simulink model "Model"  (R2019a)
settings: configuration reference "Configuration" (kept outside this file)
undefined symbols (not defined in the file): DiscIntNeverNeededParam
libraries: AP_Math x3, Quaternion x2
settings Model: Creator=zouji  LastModifiedBy=Bingo
settings ConfigSetRef: SourceName=Configuration  SourceLocation=Base Workspace

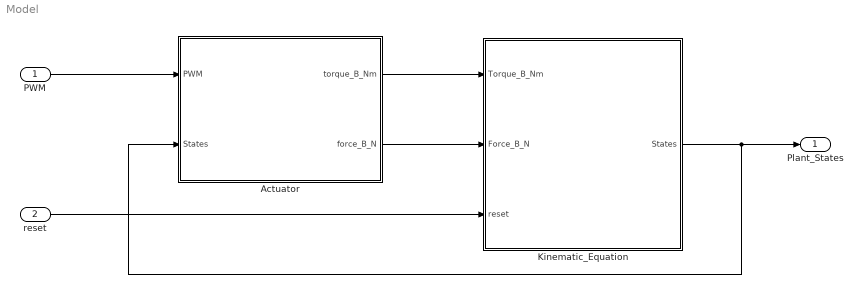
== system Model ==
  PWM : Inport
  reset : Inport  Port=2
  Actuator : Subsystem
  Kinematic_Equation : Subsystem
  Plant_States : Outport  OutDataTypeStr=Bus: Plant_States
  wires:
  Kinematic_Equation/1(States) -> Plant_States/1, Actuator/2(States)
  PWM/1 -> Actuator/1(PWM)
  Actuator/1(torque_B_Nm) -> Kinematic_Equation/1(Torque_B_Nm)
  Actuator/2(force_B_N) -> Kinematic_Equation/2(Force_B_N)
  reset/1 -> Kinematic_Equation/3(reset)

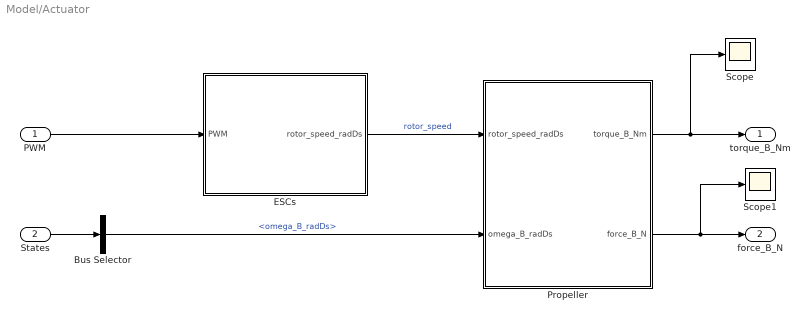
== system Model/Actuator ==
  PWM : Inport
  States : Inport  Port=2
  Bus Selector : BusSelector  OutputSignals=omega_B_radDs
  ESCs : Subsystem  mask{T=0.025, k=718.078, p=88.448}
  Propeller : Subsystem
  Scope : Scope
  Scope1 : Scope
  torque_B_Nm : Outport
  force_B_N : Outport  Port=2
  wires:
  PWM/1 -> ESCs/1(PWM)
  States/1 -> Bus Selector/1
  Bus Selector/1 -> Propeller/2(omega_B_radDs)  "<omega_B_radDs>"
  Propeller/1(torque_B_Nm) -> Scope/1, torque_B_Nm/1
  Propeller/2(force_B_N) -> Scope1/1, force_B_N/1
  ESCs/1(rotor_speed_radDs) -> Propeller/1(rotor_speed_radDs)  "rotor_speed"

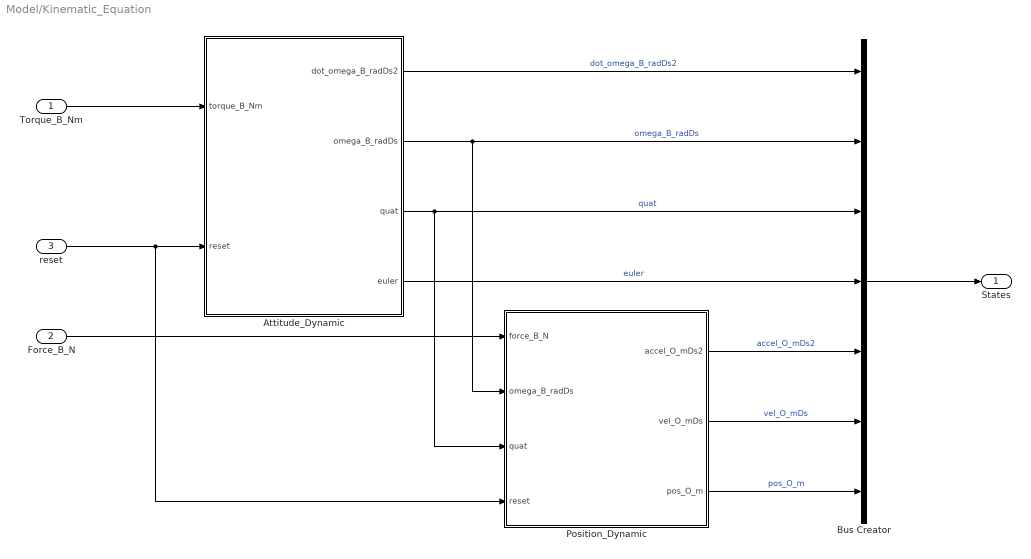
== system Model/Kinematic_Equation ==
  Torque_B_Nm : Inport
  Force_B_N : Inport  Port=2
  reset : Inport  Port=3
  Attitude_Dynamic : Subsystem  mask{Ixx=0.016, Iyy=0.016, Izz=0.0274}
  Bus Creator : BusCreator  Inputs=7
  Position_Dynamic : Subsystem  mask{mass=0.886}
  States : Outport
  wires:
  Torque_B_Nm/1 -> Attitude_Dynamic/1(torque_B_Nm)
  Force_B_N/1 -> Position_Dynamic/1(force_B_N)
  Attitude_Dynamic/2(omega_B_radDs) -> Bus Creator/2, Position_Dynamic/2(omega_B_radDs)  "omega_B_radDs"
  Attitude_Dynamic/3(quat) -> Bus Creator/3, Position_Dynamic/3(quat)  "quat"
  reset/1 -> Position_Dynamic/4(reset), Attitude_Dynamic/2(reset)
  Bus Creator/1 -> States/1
  Attitude_Dynamic/1(dot_omega_B_radDs2) -> Bus Creator/1  "dot_omega_B_radDs2"
  Attitude_Dynamic/4(euler) -> Bus Creator/4  "euler"
  Position_Dynamic/1(accel_O_mDs2) -> Bus Creator/5  "accel_O_mDs2"
  Position_Dynamic/2(vel_O_mDs) -> Bus Creator/6  "vel_O_mDs"
  Position_Dynamic/3(pos_O_m) -> Bus Creator/7  "pos_O_m"

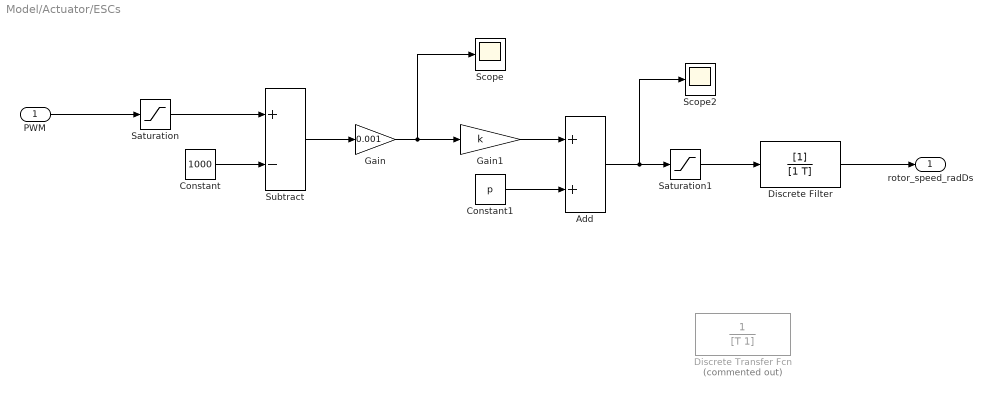
== system Model/Actuator/ESCs ==
  PWM : Inport
  Add : Sum
  Constant : Constant  Value=1000  OutDataTypeStr=uint16
  Constant1 : Constant  Value=p  OutDataTypeStr=single
  Discrete Transfer Fcn : DiscreteTransferFcn  Commented=on  Denominator=[T 1]  OutDataTypeStr=Inherit: Same as input
  Discrete Filter : DiscreteFilter  Denominator=[1 T]
  Gain : Gain  Gain=0.001  OutDataTypeStr=single
  Gain1 : Gain  Gain=k  OutDataTypeStr=Inherit: Same as input
  Saturation : Saturate  UpperLimit=2000  LowerLimit=1000
  Saturation1 : Saturate  UpperLimit=9999999  LowerLimit=0
  Scope : Scope
  Scope2 : Scope
  Subtract : Sum  Inputs=+-  OutDataTypeStr=Inherit: Same as accumulator
  rotor_speed_radDs : Outport
  wires:
  PWM/1 -> Saturation/1
  Constant/1 -> Subtract/2
  Subtract/1 -> Gain/1
  Gain/1 -> Scope/1, Gain1/1
  Gain1/1 -> Add/1
  Constant1/1 -> Add/2
  Add/1 -> Saturation1/1, Scope2/1
  Saturation/1 -> Subtract/1
  Discrete Filter/1 -> rotor_speed_radDs/1
  Saturation1/1 -> Discrete Filter/1

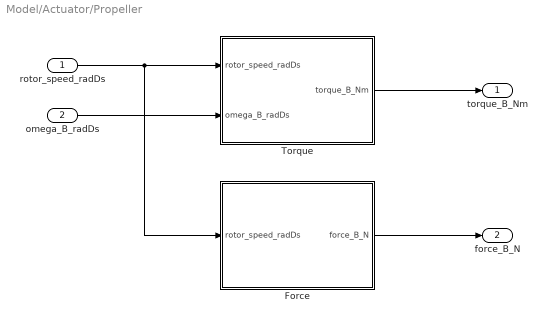
== system Model/Actuator/Propeller ==
  rotor_speed_radDs : Inport
  omega_B_radDs : Inport  Port=2
  Force : Subsystem
  Torque : Subsystem
  torque_B_Nm : Outport
  force_B_N : Outport  Port=2
  wires:
  rotor_speed_radDs/1 -> Force/1(rotor_speed_radDs), Torque/1(rotor_speed_radDs)
  Force/1(force_B_N) -> force_B_N/1
  Torque/1(torque_B_Nm) -> torque_B_Nm/1
  omega_B_radDs/1 -> Torque/2(omega_B_radDs)

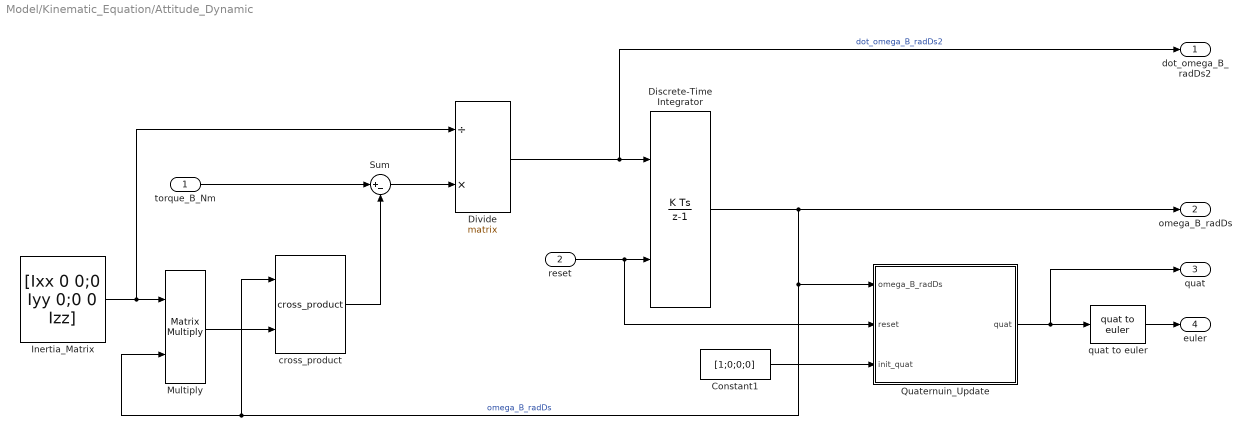
== system Model/Kinematic_Equation/Attitude_Dynamic ==
  torque_B_Nm : Inport
  reset : Inport  Port=2
  Constant1 : Constant  Value=[1;0;0;0]  OutDataTypeStr=single
  Discrete-Time Integrator : DiscreteIntegrator  ExternalReset=level  InitialCondition=[0;0;0]  SampleTime=-1  ICPrevOutput=DiscIntNeverNeededParam  ICPrevScaledInput=DiscIntNeverNeededParam
  Divide : Product  Inputs=/*  Multiplication=Matrix(*)  OutDataTypeStr=Inherit: Same as first input
  Inertia_Matrix : Constant  Value=[Ixx 0 0;0 Iyy 0;0 0 Izz]  OutDataTypeStr=single
  Multiply : Product  Multiplication=Matrix(*)  OutDataTypeStr=Inherit: Same as first input
  Quaternuin_Update : Subsystem
  Sum : Sum  Inputs=|+-  OutDataTypeStr=Inherit: Same as first input
  cross_product : AP_Math/cross_product  SystemSampleTime=-1
  quat to euler : Quaternion/quat to euler  SystemSampleTime=-1
  dot_omega_B_radDs2 : Outport
  omega_B_radDs : Outport  Port=2
  quat : Outport  Port=3
  euler : Outport  Port=4
  wires:
  Discrete-Time Integrator/1 -> Quaternuin_Update/1(omega_B_radDs), cross_product/1, Multiply/2, omega_B_radDs/1  "omega_B_radDs"
  Inertia_Matrix/1 -> Divide/1, Multiply/1
  Multiply/1 -> cross_product/2
  torque_B_Nm/1 -> Sum/1
  cross_product/1 -> Sum/2
  Sum/1 -> Divide/2
  Divide/1 -> Discrete-Time Integrator/1, dot_omega_B_radDs2/1  "dot_omega_B_radDs2"
  reset/1 -> Discrete-Time Integrator/2, Quaternuin_Update/2(reset)
  Quaternuin_Update/1(quat) -> quat/1, quat to euler/1
  quat to euler/1 -> euler/1
  Constant1/1 -> Quaternuin_Update/3(init_quat)

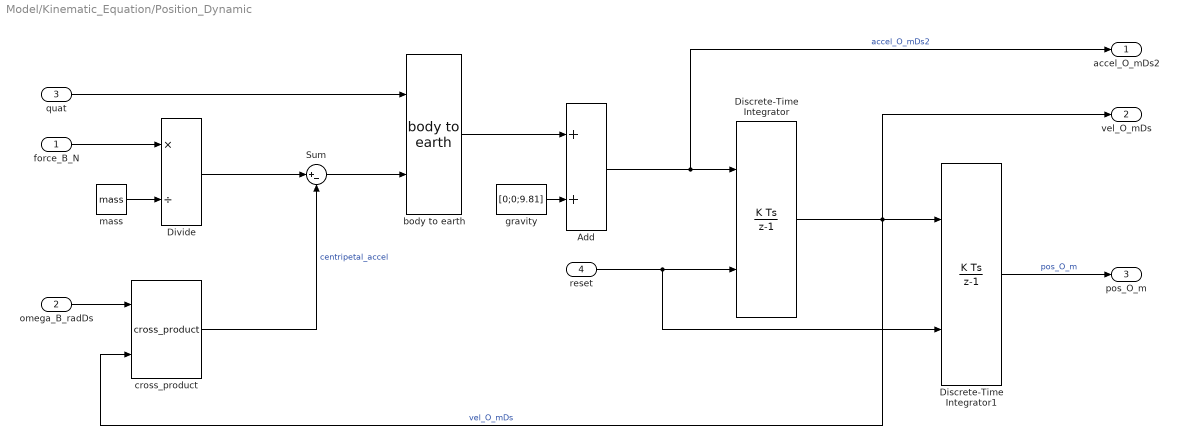
== system Model/Kinematic_Equation/Position_Dynamic ==
  force_B_N : Inport
  omega_B_radDs : Inport  Port=2
  quat : Inport  Port=3
  reset : Inport  Port=4
  Add : Sum
  Discrete-Time Integrator : DiscreteIntegrator  ExternalReset=level  InitialCondition=[0;0;0]  SampleTime=-1  ICPrevOutput=DiscIntNeverNeededParam  ICPrevScaledInput=DiscIntNeverNeededParam
  Discrete-Time Integrator1 : DiscreteIntegrator  ExternalReset=level  InitialCondition=[0;0;0]  SampleTime=-1  ICPrevOutput=DiscIntNeverNeededParam  ICPrevScaledInput=DiscIntNeverNeededParam
  Divide : Product  Inputs=*/
  Sum : Sum  Inputs=|+-
  body to earth : Quaternion/body to earth  SystemSampleTime=-1
  cross_product : AP_Math/cross_product  SystemSampleTime=-1
  gravity : Constant  Value=[0;0;9.81]  OutDataTypeStr=single
  mass : Constant  Value=mass  OutDataTypeStr=single
  accel_O_mDs2 : Outport
  vel_O_mDs : Outport  Port=2
  pos_O_m : Outport  Port=3
  wires:
  force_B_N/1 -> Divide/1
  mass/1 -> Divide/2
  Discrete-Time Integrator/1 -> cross_product/2, Discrete-Time Integrator1/1, vel_O_mDs/1  "vel_O_mDs"
  omega_B_radDs/1 -> cross_product/1
  Divide/1 -> Sum/1
  cross_product/1 -> Sum/2  "centripetal_accel"
  Sum/1 -> body to earth/2
  quat/1 -> body to earth/1
  body to earth/1 -> Add/1
  gravity/1 -> Add/2
  Add/1 -> accel_O_mDs2/1, Discrete-Time Integrator/1  "accel_O_mDs2"
  reset/1 -> Discrete-Time Integrator1/2, Discrete-Time Integrator/2
  Discrete-Time Integrator1/1 -> pos_O_m/1  "pos_O_m"

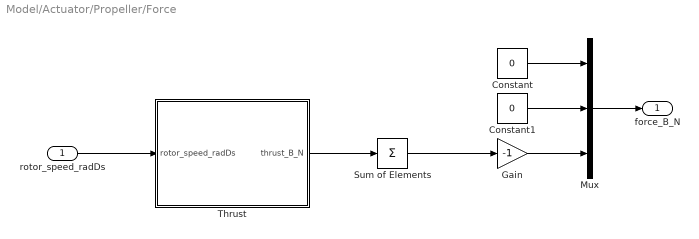
== system Model/Actuator/Propeller/Force ==
  rotor_speed_radDs : Inport
  Constant : Constant  Value=0  OutDataTypeStr=single
  Constant1 : Constant  Value=0  OutDataTypeStr=single
  Gain : Gain  Gain=-1  OutDataTypeStr=Inherit: Same as input
  Mux : Mux  Inputs=3
  Sum of Elements : Sum  Inputs=+
  Thrust : Subsystem  mask{cT=1.239e-5}
  force_B_N : Outport
  wires:
  rotor_speed_radDs/1 -> Thrust/1(rotor_speed_radDs)
  Sum of Elements/1 -> Gain/1
  Thrust/1(thrust_B_N) -> Sum of Elements/1
  Gain/1 -> Mux/3
  Mux/1 -> force_B_N/1
  Constant/1 -> Mux/1
  Constant1/1 -> Mux/2

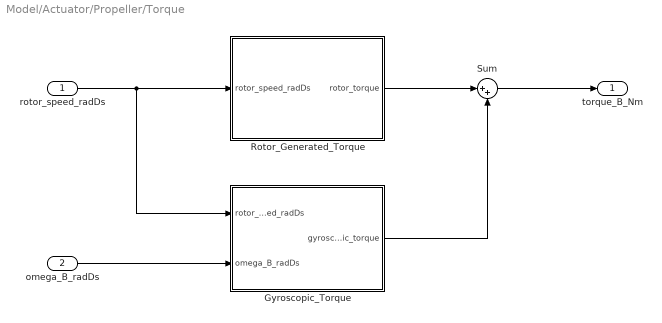
== system Model/Actuator/Propeller/Torque ==
  rotor_speed_radDs : Inport
  omega_B_radDs : Inport  Port=2
  Gyroscopic_Torque : Subsystem  mask{Im=3.789e-6}
  Rotor_Generated_Torque : Subsystem  mask{L=0.255*sin(pi/4), cT=1.23884e-5, cQ=1.982e-7}
  Sum : Sum  Inputs=|++
  torque_B_Nm : Outport
  wires:
  rotor_speed_radDs/1 -> Gyroscopic_Torque/1(rotor_speed_radDs), Rotor_Generated_Torque/1(rotor_speed_radDs)
  omega_B_radDs/1 -> Gyroscopic_Torque/2(omega_B_radDs)
  Rotor_Generated_Torque/1(rotor_torque) -> Sum/1
  Sum/1 -> torque_B_Nm/1
  Gyroscopic_Torque/1(gyroscopic_torque) -> Sum/2

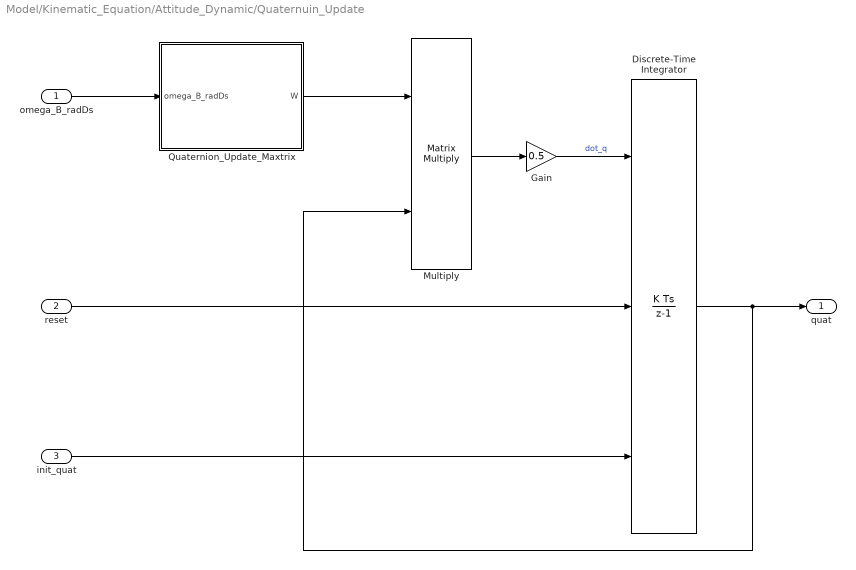
== system Model/Kinematic_Equation/Attitude_Dynamic/Quaternuin_Update ==
  omega_B_radDs : Inport
  reset : Inport  Port=2
  init_quat : Inport  Port=3
  Discrete-Time Integrator : DiscreteIntegrator  ExternalReset=level  InitialConditionSource=external  SampleTime=-1  ICPrevOutput=DiscIntNeverNeededParam  ICPrevScaledInput=DiscIntNeverNeededParam
  Gain : Gain  Gain=0.5  OutDataTypeStr=Inherit: Same as input
  Multiply : Product  Multiplication=Matrix(*)  OutDataTypeStr=Inherit: Same as first input
  Quaternion_Update_Maxtrix : Subsystem
  quat : Outport
  wires:
  omega_B_radDs/1 -> Quaternion_Update_Maxtrix/1(omega_B_radDs)
  Quaternion_Update_Maxtrix/1(W) -> Multiply/1
  Multiply/1 -> Gain/1
  reset/1 -> Discrete-Time Integrator/2
  init_quat/1 -> Discrete-Time Integrator/3
  Discrete-Time Integrator/1 -> Multiply/2, quat/1
  Gain/1 -> Discrete-Time Integrator/1  "dot_q"

== system Model/Actuator/Propeller/Force/Thrust ==
  rotor_speed_radDs : Inport
  Multiply : Product  OutDataTypeStr=Inherit: Same as first input
  Square : Math  Operator=square  SaturateOnIntegerOverflow=on
  cT : Constant  Value=cT
  thrust_B_N : Outport
  wires:
  rotor_speed_radDs/1 -> Square/1
  Square/1 -> Multiply/1
  cT/1 -> Multiply/2
  Multiply/1 -> thrust_B_N/1

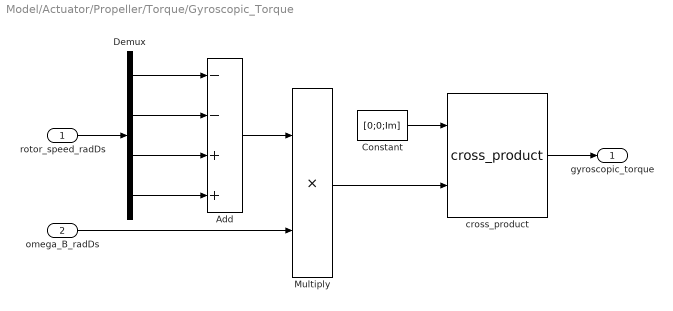
== system Model/Actuator/Propeller/Torque/Gyroscopic_Torque ==
  rotor_speed_radDs : Inport
  omega_B_radDs : Inport  Port=2
  Add : Sum  Inputs=--++
  Constant : Constant  Value=[0;0;Im]  OutDataTypeStr=single
  Demux : Demux
  Multiply : Product
  cross_product : AP_Math/cross_product  SystemSampleTime=-1
  gyroscopic_torque : Outport
  wires:
  Demux/1 -> Add/1
  Constant/1 -> cross_product/1
  Demux/4 -> Add/4
  Add/1 -> Multiply/1
  Demux/3 -> Add/3
  Demux/2 -> Add/2
  omega_B_radDs/1 -> Multiply/2
  Multiply/1 -> cross_product/2
  cross_product/1 -> gyroscopic_torque/1
  rotor_speed_radDs/1 -> Demux/1

== system Model/Actuator/Propeller/Torque/Rotor_Generated_Torque ==
  rotor_speed_radDs : Inport
  Multiply : Product  Multiplication=Matrix(*)
  Square : Math  Operator=square  SaturateOnIntegerOverflow=on
  X_Frame : Constant  Value=[-L*cT,L*cT,L*cT,-L*cT;L*cT,-L*cT,L*cT,-L*cT;cQ,cQ,-cQ,-cQ]  OutDataTypeStr=single
  rotor_torque : Outport
  wires:
  X_Frame/1 -> Multiply/1
  Square/1 -> Multiply/2
  Multiply/1 -> rotor_torque/1
  rotor_speed_radDs/1 -> Square/1

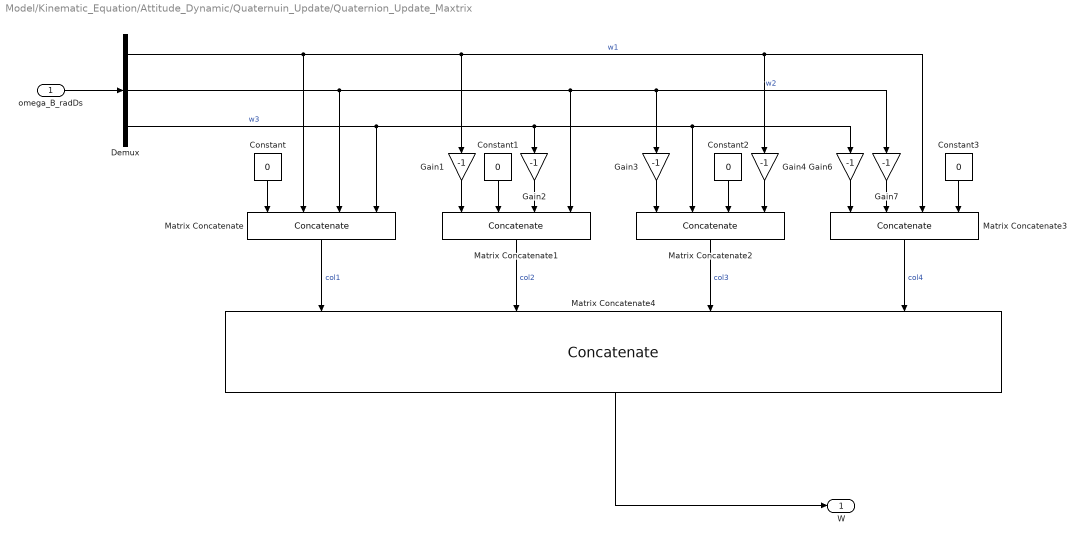
== system Model/Kinematic_Equation/Attitude_Dynamic/Quaternuin_Update/Quaternion_Update_Maxtrix ==
  omega_B_radDs : Inport
  Constant{,1..3} (4 alike) : Constant  Value=0  OutDataTypeStr=single
  Demux : Demux  Outputs=3
  Gain{1..4,6..7} (6 alike) : Gain  Gain=-1  OutDataTypeStr=Inherit: Same as input
  Matrix Concatenate{,1..3} (4 alike) : Concatenate  NumInputs=4
  Matrix Concatenate4 : Concatenate  NumInputs=4  Mode=Multidimensional array  ConcatenateDimension=2
  W : Outport
  wires:
  Gain4/1 -> Matrix Concatenate2/4
  omega_B_radDs/1 -> Demux/1
  Gain2/1 -> Matrix Concatenate1/3
  Demux/3 -> Matrix Concatenate/4, Matrix Concatenate2/2, Gain6/1, Gain2/1  "w3"
  Gain3/1 -> Matrix Concatenate2/1
  Constant/1 -> Matrix Concatenate/1
  Demux/2 -> Matrix Concatenate/3, Matrix Concatenate1/4, Gain7/1, Gain3/1  "w2"
  Matrix Concatenate3/1 -> Matrix Concatenate4/4  "col4"
  Constant1/1 -> Matrix Concatenate1/2
  Gain6/1 -> Matrix Concatenate3/1
  Constant3/1 -> Matrix Concatenate3/4
  Matrix Concatenate1/1 -> Matrix Concatenate4/2  "col2"
  Matrix Concatenate/1 -> Matrix Concatenate4/1  "col1"
  Demux/1 -> Matrix Concatenate/2, Matrix Concatenate3/3, Gain4/1, Gain1/1  "w1"
  Matrix Concatenate4/1 -> W/1
  Constant2/1 -> Matrix Concatenate2/3
  Matrix Concatenate2/1 -> Matrix Concatenate4/3  "col3"
  Gain7/1 -> Matrix Concatenate3/2
  Gain1/1 -> Matrix Concatenate1/1
